simulink model "zad1"  (R2018a)
settings: Solver=VariableStepAuto  StartTime=0.0  StopTime=25  RelTol=1e-3
settings Model: Creator=Koala  LastModifiedBy=Koala

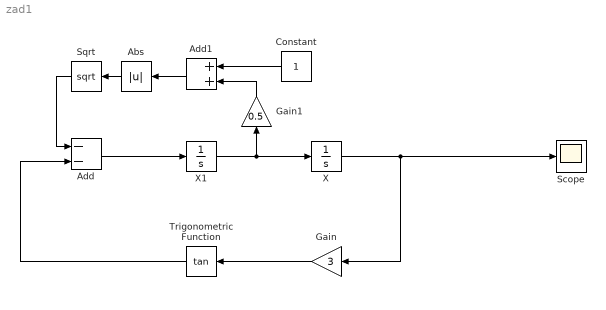
== system zad1 ==
  Abs : Abs
  Add : Sum  Inputs=--
  Add1 : Sum
  Constant : Constant
  Gain : Gain  Gain=3
  Gain1 : Gain  Gain=0.5
  Scope : Scope
  Sqrt : Sqrt  SaturateOnIntegerOverflow=on
  Trigonometric Function : Trigonometry  Operator=tan
  "X " : Integrator  InitialCondition=1
  "X1 " : Integrator
  wires:
  "X1 "/1 -> Gain1/1, "X "/1
  "X "/1 -> Scope/1, Gain/1
  Gain/1 -> Trigonometric Function/1
  Trigonometric Function/1 -> Add/2
  Add/1 -> "X1 "/1
  Constant/1 -> Add1/1
  Add1/1 -> Abs/1
  Abs/1 -> Sqrt/1
  Sqrt/1 -> Add/1
  Gain1/1 -> Add1/2
